simulink model "level1"  (R2018a)
settings: Solver=VariableStepAuto  StartTime=0.0  StopTime=10.0  RelTol=1e-3
settings Model: Creator=gonzalo  LastModifiedBy=gonzalo

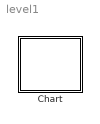
== system level1 ==
  Chart : Stateflow chart  TreatAsAtomicUnit=on

== stateflow chart level1/Chart ==
  state Level1
    state Start [parallel]
      settings: executionOrder=1
      state Manual
        entry:
        during:
      state Automatico
        entry:
        during:
      (default) -> Manual
      Manual -> Automatico : [automatic == 1]
      Automatico -> Manual : [automatic == 0]
    state Spreader [parallel]
      settings: executionOrder=2
      state Charged
      state Unchaged
      (default) -> Charged
      Charged -> Unchaged : [twistlocks == 0]
      Unchaged -> Charged : [twistlocks == 1]
    state Balancing_Control [parallel]
      settings: executionOrder=3
      state Activated
      state Disactivated
      (default) -> Activated
      Activated -> Disactivated : [balacing_control == 0]
      Disactivated -> Activated : [balancing_control == 1]
  (default) -> Level1
